simulink model "ADC_reader_simulink"  (R2025a)
settings: Solver=FixedStepAuto  StartTime=0.0  StopTime=inf  RelTol=1e-3  EnableMultiTasking=on
libraries: stm32f4xxblockslib x10, dspfdesign x1, dspstat3 x1
settings Model: STM32="{\"AnalogInput\":[{\"ID\":\"test_poten:20\"},{\"ID\":\"test_poten:28\"},{\"ID\":\"ADC_reader:28\"},{\"ID\":\"ADC_reader:20\"},{\"ID\":\"ADC_reader:14\"},{\"ID\":\"ADC_reader:11\"},{\"ID\":\"ADC_reader:8\"},{\"ID\":\"ADC_reader:5\"},{\"ID\":\"ADC_reader:1\"},{\"ID\":\"ADC_reader_simulink:14\"},{\"ID\":\"ADC_reader_simulink:11\"},{\"ID\":\"ADC_reader_simulink:8\"},{\"ID\":\"ADC_reader_simulink:5\"},{\"ID\":\"ADC_reader_simulink:1\"},{\"ID\":\"ADC_reader_simulink:86\"},{\"ID\":\"ADC_reader_simulink:111\"},{\"ID\":\"ADC_reader_simulink:20\"},{\"ID\":\"ADC_reader_simulink:125\"}]}"  Creator=ioonz  LastModifiedBy=POND
settings OptimizationCC: DefaultParameterBehavior=Inlined  EnhancedBackFolding=on  PassReuseOutputArgsAs=Individual arguments  ZeroExternalMemoryAtStartup=off  ZeroInternalMemoryAtStartup=off  MaxStackSize=512  OptimizeBlockOrder=speed  DifferentSizesBufferReuse=on  OptimizationCustomize=off  EfficientTunableParamExpr=on
settings DebuggingCC: ParameterTunabilityLossMsg=error
settings HardwareCC: ProdBitPerPointer=32.0  ProdBitPerSizeT=32.0  ProdBitPerPtrDiffT=32.0  ProdLargestAtomicInteger=Long  ProdLargestAtomicFloat=Double  ProdWordSize=32.0  ProdLongLongMode=on  ProdHWDeviceType=ARM Compatible->ARM Cortex-M
settings SFSimCC: MATLABDynamicMemAlloc=off
settings RTWCC: SystemTargetFile=ert.tlc  HardwareBoard=STM32G4xx Based  TemplateMakefile=ert_default_tmf  Toolchain=GNU Tools for ARM Embedded Processors  Description=Embedded Coder
settings CodeAppCC: ForceParamTrailComments=on  IgnoreCustomStorageClasses=off  OperatorAnnotations=on  SimulinkDataObjDesc=on  SFDataObjDesc=on  InsertBlockDesc=on
settings ERTTargetCC: ExtModeTransport=3.0  ExtModeStaticAllocSize=2048.0  TargetLangStandard=C99 (ISO)  CodeReplacementLibrary=ARM Cortex-M

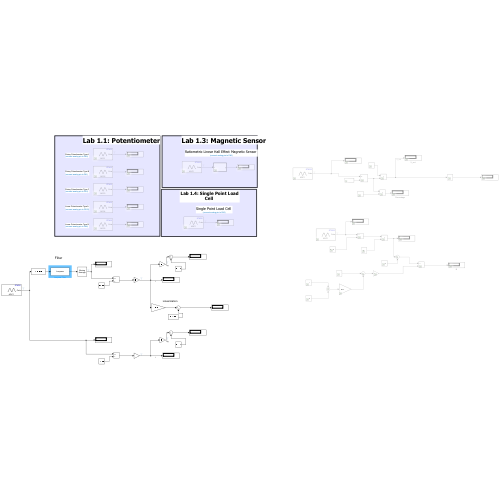
[thumbnail: Simulink's stored preview of the top-level diagram]
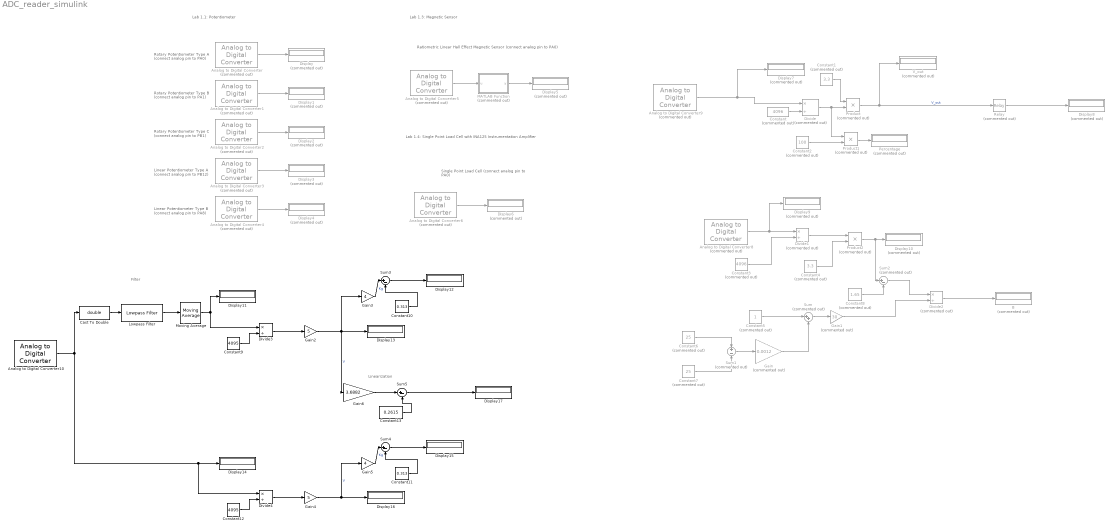
== system ADC_reader_simulink ==
  note: Linearization
  note: Lab 1.1: Potentiometer
  note: Rotary Potentiometer Type A
      | (connect analog pin to PA0)
  note: Rotary Potentiometer Type B
      | (connect analog pin to PA1)
  note: Rotary Potentiometer Type C
      | (connect analog pin to PB1)
  note: Linear Potentiometer Type A
      | (connect analog pin to PB12)
  note: Linear Potentiometer Type B
      | (connect analog pin to PA8)
  note: Ratiometric Linear Hall Effect Magnetic Sensor
      | (connect analog pin to PA0)
  note: Single Point Load Cell
      | (connect analog pin to PA0)
  note: Lab 1.3: Magnetic Sensor
  note: Lab 1.4: Single Point Load Cell
      | with INA125 Instrumentation Amplifier
  note: Filter
  Analog to Digital Converter{,5..6,8..9} (5 alike) : stm32f4xxblockslib/Analog to Digital Converter  Commented=on  ADCModule=ADC1  ConversionGroup=Regular  TriggerMode=Trigger and read  NumberOfConversions=1  EnableBufferConv=off  BufferLength=1  OutputStatus=off  SampleTime=-1  EnableSimPort=off  hoistedMaskSrc=ECSoC/ECSimCodegen/Analog to Digital Converter
  Analog to Digital Converter1 : stm32f4xxblockslib/Analog to Digital Converter  Commented=on  ADCModule=ADC2  ConversionGroup=Regular  TriggerMode=Trigger and read  NumberOfConversions=1  EnableBufferConv=off  BufferLength=1  OutputStatus=off  SampleTime=-1  EnableSimPort=off  hoistedMaskSrc=ECSoC/ECSimCodegen/Analog to Digital Converter
  Analog to Digital Converter10 : stm32f4xxblockslib/Analog to Digital Converter  ADCModule=ADC1  ConversionGroup=Regular  TriggerMode=Trigger and read  NumberOfConversions=1  EnableBufferConv=off  BufferLength=1  OutputStatus=off  SampleTime=0.01  EnableSimPort=off  hoistedMaskSrc=ECSoC/ECSimCodegen/Analog to Digital Converter
  Analog to Digital Converter2 : stm32f4xxblockslib/Analog to Digital Converter  Commented=on  ADCModule=ADC3  ConversionGroup=Regular  TriggerMode=Trigger and read  NumberOfConversions=1  EnableBufferConv=off  BufferLength=1  OutputStatus=off  SampleTime=-1  EnableSimPort=off  hoistedMaskSrc=ECSoC/ECSimCodegen/Analog to Digital Converter
  Analog to Digital Converter3 : stm32f4xxblockslib/Analog to Digital Converter  Commented=on  ADCModule=ADC4  ConversionGroup=Regular  TriggerMode=Trigger and read  NumberOfConversions=1  EnableBufferConv=off  BufferLength=1  OutputStatus=off  SampleTime=-1  EnableSimPort=off  hoistedMaskSrc=ECSoC/ECSimCodegen/Analog to Digital Converter
  Analog to Digital Converter4 : stm32f4xxblockslib/Analog to Digital Converter  Commented=on  ADCModule=ADC5  ConversionGroup=Regular  TriggerMode=Trigger and read  NumberOfConversions=1  EnableBufferConv=off  BufferLength=1  OutputStatus=off  SampleTime=-1  EnableSimPort=off  hoistedMaskSrc=ECSoC/ECSimCodegen/Analog to Digital Converter
  B : Display  Commented=on
  Cast To Double : DataTypeConversion  OutDataTypeStr=double  SaturateOnIntegerOverflow=off  RndMeth=Floor
  Constant : Constant  Commented=on  Value=4096
  Constant1 : Constant  Commented=on  Value=3.3
  Constant10 : Constant  Value=0.313
  Constant11 : Constant  Value=0.313
  Constant12 : Constant  Value=4095
  Constant13 : Constant  Value=0.2615
  Constant2 : Constant  Commented=on  Value=100
  Constant3 : Constant  Commented=on  Value=4096
  Constant4 : Constant  Commented=on  Value=3.3
  Constant5 : Constant  Commented=on
  Constant6 : Constant  Commented=on  Value=25
  Constant7 : Constant  Commented=on  Value=25
  Constant8 : Constant  Commented=on  Value=1.65
  Constant9 : Constant  Value=4095
  Display{,1..10} (11 alike) : Display  Commented=on
  Display{11..17} (7 alike) : Display
  Divide : Product  Commented=on  Inputs=*/
  Divide1 : Product  Commented=on  Inputs=*/
  Divide2 : Product  Commented=on  Inputs=*/
  Divide3 : Product  Inputs=*/
  Divide4 : Product  Inputs=*/
  Gain : Gain  Commented=on  Gain=0.0012
  Gain1 : Gain  Commented=on  Gain=30
  Gain2 : Gain  Gain=5
  Gain3 : Gain  Gain=4
  Gain4 : Gain  Gain=5
  Gain5 : Gain  Gain=4
  Gain6 : Gain  Gain=3.6882
  Lowpass Filter : dspfdesign/Lowpass Filter  FilterType=IIR  DesignForMinimumOrder=off  FilterOrder=4  PassbandFrequency=10  StopbandFrequency=0.5442  PassbandRipple=0.1  StopbandAttenuation=80  SampleRateMode=Specify on dialog  SampleRate=100  SimulateUsing=Interpreted execution  roundingMode=Floor  coeffsDataTypeStr=fixdt(1,16)
  MATLAB Function : MATLAB Function  Commented=on  TreatAsAtomicUnit=on
  Moving Average : dspstat3/Moving Average  Method=Sliding window  ForgettingFactorPort=off  SpecifyWindowLength=on  WindowLength=4  OverlapLength=3  AllowArbitraryInputLength=off  ForgettingFactor=0.9  SimulateUsing=Interpreted execution
  Percentage : Display  Commented=on
  Product : Product  Commented=on
  Product1 : Product  Commented=on
  Product2 : Product  Commented=on
  Relay : Relay  Commented=on  OnSwitchValue=2  OffSwitchValue=2
  Sum : Sum  Commented=on  Inputs=|++
  Sum1 : Sum  Commented=on  Inputs=+-
  Sum2 : Sum  Commented=on  Inputs=|+-
  Sum3 : Sum  Inputs=|+-
  Sum4 : Sum  Inputs=|+-
  Sum5 : Sum  Inputs=|+-
  V_out : Display  Commented=on
  wires:
  Analog to Digital Converter/1 -> Display/1
  Analog to Digital Converter1/1 -> Display1/1
  Analog to Digital Converter2/1 -> Display2/1
  Analog to Digital Converter3/1 -> Display3/1
  Analog to Digital Converter4/1 -> Display4/1
  Analog to Digital Converter5/1 -> MATLAB Function/1(u)
  Analog to Digital Converter6/1 -> Display6/1
  Constant/1 -> Divide/2
  Divide/1 -> Product1/1, Product/2
  Constant1/1 -> Product/1
  Product/1 -> Relay/1, V_out/1  "V_out"
  Relay/1 -> Display8/1
  Constant2/1 -> Product1/2
  Product1/1 -> Percentage/1
  Analog to Digital Converter9/1 -> Display7/1, Divide/1
  Analog to Digital Converter8/1 -> Divide1/1, Display9/1
  Constant3/1 -> Divide1/2
  Constant4/1 -> Product2/2
  Divide1/1 -> Product2/1
  Product2/1 -> Sum2/1, Display10/1
  Constant5/1 -> Sum/1
  Gain/1 -> Sum/2
  Constant6/1 -> Sum1/1
  Constant7/1 -> Sum1/2
  Sum1/1 -> Gain/1
  Sum/1 -> Gain1/1
  Constant8/1 -> Sum2/2
  Sum2/1 -> Divide2/1
  Gain1/1 -> Divide2/2
  Divide2/1 -> B/1
  MATLAB Function/1(y) -> Display5/1
  Constant9/1 -> Divide3/2
  Divide3/1 -> Gain2/1
  Gain2/1 -> Gain6/1, Display13/1, Gain3/1  "V"
  Gain3/1 -> Sum3/1  "Kg"
  Constant10/1 -> Sum3/2
  Sum3/1 -> Display12/1
  Lowpass Filter/1 -> Moving Average/1
  Constant12/1 -> Divide4/2
  Divide4/1 -> Gain4/1
  Gain4/1 -> Display16/1, Gain5/1  "V"
  Gain5/1 -> Sum4/1  "Kg"
  Constant11/1 -> Sum4/2
  Sum4/1 -> Display15/1
  Analog to Digital Converter10/1 -> Cast To Double/1, Divide4/1, Display14/1
  Moving Average/1 -> Divide3/1, Display11/1
  Cast To Double/1 -> Lowpass Filter/1
  Gain6/1 -> Sum5/1
  Constant13/1 -> Sum5/2
  Sum5/1 -> Display17/1

== matlab function ADC_reader_simulink/MATLAB Function ==
  data: u input; y output
function y = averageFilter(u)
% u : ค่าที่อ่านได้จากเซ็นเซอร์ (input)
% y : ค่าที่เฉลี่ยแล้ว (output)

persistent buffer index count
N = 1000;  % จำนวนค่าที่จะใช้ในการเฉลี่ย

% สร้างตัวแปร persistent ครั้งแรก
if isempty(buffer)
    buffer = zeros(1, N);
    index = 1;
    count = 0;
end

% เก็บค่าล่าสุดลงใน buffer
buffer(index) = u;
index = index + 1;

% วนกลับไปที่ตำแหน่งแรกเมื่อครบ N ค่า
if index > N
    index = 1;
end

% นับจำนวนค่าที่เก็บ (ไม่เกิน N)
if count < N
    count = count + 1;
end

% คำนวณค่าเฉลี่ย
y = sum(buffer) / count;
